simulink model "sf_tlevery"  (Simulink 7.6)
settings: Solver=ode45  StartTime=0.0  StopTime=100  RelTol=1e-3
settings Model: Creator=The MathWorks Inc.  CovMetricSettings=dcmtr  ExtModeAutoUpdateStatusClock=off
settings OptimizationCC: BooleanDataType=off  InlineInvariantSignals=on  InitFltsAndDblsToZero=on  EfficientMapNaN2IntZero=off
settings DebuggingCC: SaveWithParameterizedLinksMsg=none  SignalResolutionControl=TryResolveAllWithWarning  SolverPrmCheckMsg=none  MultiTaskDSMMsg=warning  MultiTaskCondExecSysMsg=none  StrictBusMsg=None
settings HardwareCC: TargetUnknown=on
settings SFSimCC: SimParseCustomCode=off
settings RTWCC: IncludeERTFirstTime=on
settings GRTTargetCC: TargetFcnLib=ansi_tfl_tmw.mat

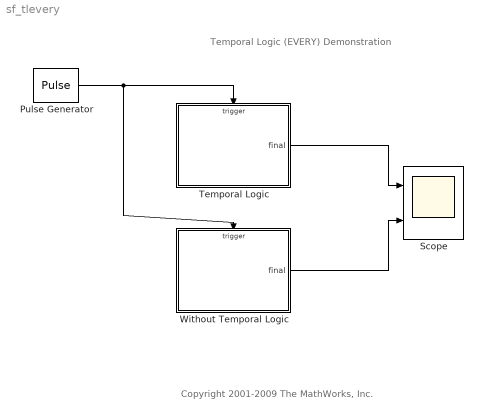
== system sf_tlevery ==
  note: Temporal Logic (EVERY) Demonstration
  note: Copyright 2001-2009 The MathWorks, Inc.
  Pulse Generator : DiscretePulseGenerator  PulseType=Time based  Period=1  PulseWidth=.5
  Scope : Scope  NumInputPorts=2
      settings: TimeRange=100  YMin=-5~-5  YMax=40~40
  Temporal Logic : Stateflow chart  TreatAsAtomicUnit=on
  Without Temporal Logic : Stateflow chart  TreatAsAtomicUnit=on
  wires:
  Pulse Generator/1 -> Temporal Logic/Trigger, Without Temporal Logic/Trigger
  Temporal Logic/1(final) -> Scope/1
  Without Temporal Logic/1(final) -> Scope/2

== stateflow chart Without Temporal Logic ==
  state Counter [parallel]
    settings: executionOrder=4
    state One
      count=1;
      One -> One : {count++;}
  state State [parallel]
    settings: executionOrder=1
    state A
    A -> (junction 12) : [count==5]{first_counter++;}
    (junction 12) -> A : {count=0;}
  state output = double_counter(input) [function]
    (default) -> (junction 13) : {output=2*input;}
  state State_two [parallel]
    settings: executionOrder=2
    state B
    B -> (junction 14) : [n==10]{final=double_counter(first_counter);}
    (junction 14) -> B : {n=0;}
  state Counter_two [parallel]
    settings: executionOrder=3
    state Two
      n=1;
      Two -> Two : {n++;}
  (default) -> A : {first_counter=0;}
  data: input function_input double; output function_output double; count local double; final output double; first_counter local double; n local double
  events: secs input RISING_EDGE_EVENT

== stateflow chart Temporal Logic ==
  state output = double_counter(input) [function]
    (default) -> (junction 34) : {output=2*input;}
  state Active
    on every(5,secs): count++;
    on every(10,secs):final=double_counter(count);
  (default) -> Active : {count=0;}
  data: input function_input double; output function_output double; count local double; final output double
  events: secs input RISING_EDGE_EVENT
